simulink model "Pendel"  (R2014b)
settings: Solver=ode45  StartTime=0.0  StopTime=10.0  RelTol=1e-3
libraries: vrlib x2
settings Model: Creator=Florian  LastModifiedBy=Florian

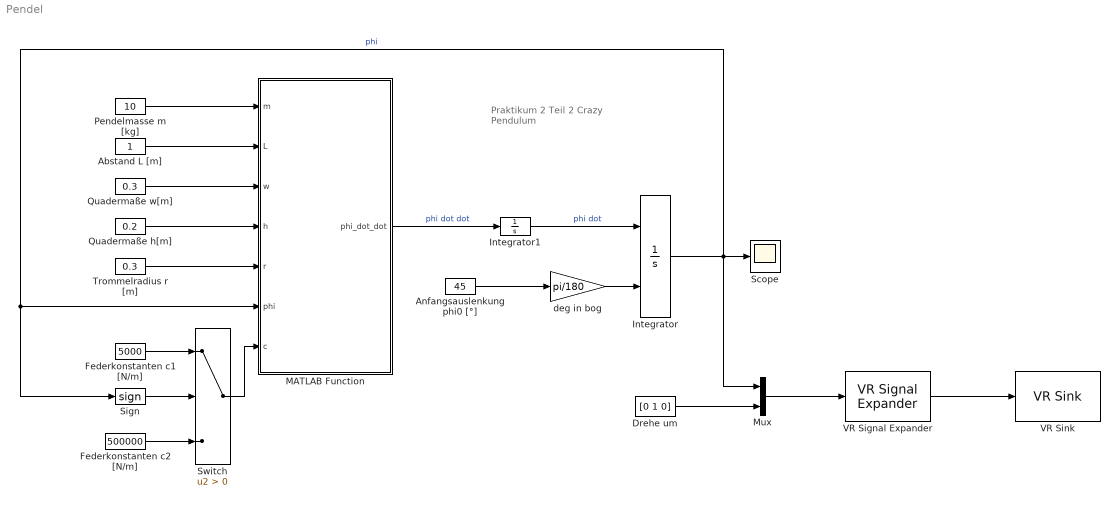
== system Pendel ==
  note: Praktikum 2
      | Teil 2
      | Crazy Pendulum
  Abstand L [m] : Constant
  Anfangsauslenkung phi0 [°] : Constant  Value=45
  "Drehe um " : Constant  Value=[0 1 0]
  Federkonstanten c1 [N/m] : Constant  Value=5000
  Federkonstanten c2 [N/m] : Constant  Value=500000
  Integrator : Integrator  InitialConditionSource=external
  Integrator1 : Integrator
  MATLAB Function : MATLAB Function  TreatAsAtomicUnit=on
  Mux : Mux  Inputs=2
  Pendelmasse m [kg] : Constant  Value=10
  Quadermaße h[m] : Constant  Value=0.2
  Quadermaße w[m] : Constant  Value=0.3
  Scope : Scope
  Sign : Signum
  Switch : Switch  Criteria=u2 > Threshold
  Trommelradius r [m] : Constant  Value=0.3
  VR Signal Expander : vrlib/VR Signal Expander  outwidth=4  outidx=[4 1 2 3]
  VR Sink : vrlib/VR Sink  InstantiateOnLoad=on  SampleTime=0.005  ViewEnable=on  RemoteChange=off  RemoteView=off  FieldsWritten=Seiltrommel.rotation.4.1.1.double  WorldFileName=gegeben\CrazyPendlm.wrl  AutoView=off  VideoDimensions=[]  AllowVariableSize=off
  deg in bog : Gain  Gain=pi/180
  wires:
  Pendelmasse m [kg]/1 -> MATLAB Function/1(m)
  Abstand L [m]/1 -> MATLAB Function/2(L)
  Quadermaße w[m]/1 -> MATLAB Function/3(w)
  Quadermaße h[m]/1 -> MATLAB Function/4(h)
  Trommelradius r [m]/1 -> MATLAB Function/5(r)
  Sign/1 -> Switch/2
  Switch/1 -> MATLAB Function/7(c)
  Federkonstanten c1 [N/m]/1 -> Switch/1
  Federkonstanten c2 [N/m]/1 -> Switch/3
  Integrator/1 -> MATLAB Function/6(phi), Sign/1, Scope/1, Mux/1  "phi"
  MATLAB Function/1(phi_dot_dot) -> Integrator1/1  "phi dot dot"
  Anfangsauslenkung phi0 [°]/1 -> deg in bog/1
  deg in bog/1 -> Integrator/2
  Integrator1/1 -> Integrator/1  "phi dot"
  "Drehe um "/1 -> Mux/2
  Mux/1 -> VR Signal Expander/1
  VR Signal Expander/1 -> VR Sink/1

== matlab function Pendel/MATLAB Function ==
  data: m input; phi_dot_dot output; L input; w input; h input; r input; phi input; c input
function phi_dot_dot = fcn(m,L,w,h,r,phi,c)

J_s= 1/12*m * (h^2 + w^2); %Massenträgheitsmoment
J_a= J_s + m*(L+h/2)^2;    %Satz von Steiner

M_pendel= m + cos(phi) * (L+h/2);
M_feder= c * phi * r^2; 

phi_dot_dot = (-M_feder+M_pendel)/J_a;
